simulink model "springslx"  (R2022a)
settings: Solver=VariableStepAuto  StartTime=0.0  StopTime=10.0  RelTol=1e-3
model workspace (MAT data in the model file):
  m = 50
settings Model: Creator=mihai  LastModifiedBy=mihai

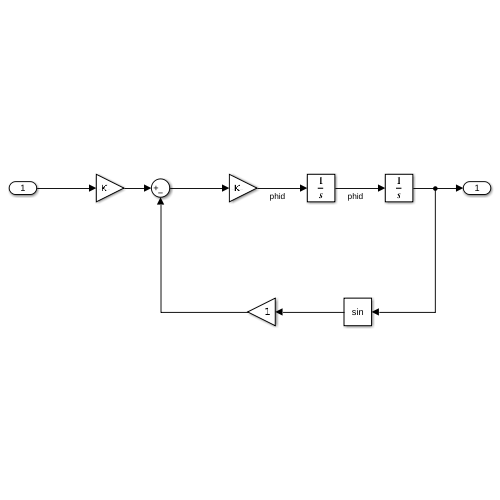
[thumbnail: Simulink's stored preview of the top-level diagram]
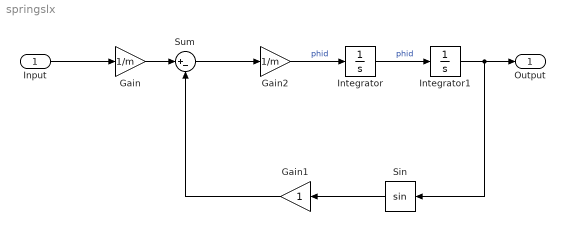
== system springslx ==
  Input : Inport
  Gain : Gain  Gain=1/m
  Gain1 : Gain
  Gain2 : Gain  Gain=1/m
  Integrator : Integrator
  Integrator1 : Integrator
  Sin : Trigonometry
  Sum : Sum  Inputs=|+-
  Output : Outport
  wires:
  Input/1 -> Gain/1
  Gain/1 -> Sum/1
  Gain1/1 -> Sum/2
  Sin/1 -> Gain1/1
  Sum/1 -> Gain2/1
  Gain2/1 -> Integrator/1  "phid"
  Integrator/1 -> Integrator1/1  "phid"
  Integrator1/1 -> Output/1, Sin/1
